simulink model "PCM"  (R2019b)
settings: Solver=FixedStepAuto  StartTime=0.0  StopTime=10.0  FixedStep=0.1  RelTol=1e-3
settings Model: Creator=JDALUZ1  LastModifiedBy=EMORAI12
settings DebuggingCC: ArithmeticOperatorsInVariantConditions=warning
settings SFSimCC: CustomCodeUndefinedFunction=UseInterfaceOnly
settings CodeAppCC: StateflowObjectComments=on

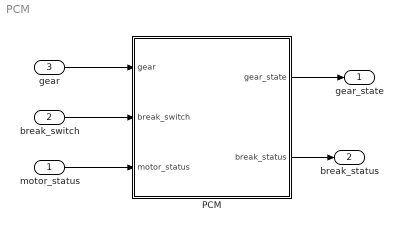
== system PCM ==
  motor_status : Inport
  break_switch : Inport  Port=2
  gear : Inport  Port=3
  PCM : Stateflow chart  TreatAsAtomicUnit=on
  gear_state : Outport
  break_status : Outport  Port=2
  wires:
  PCM/1(gear_state) -> gear_state/1
  PCM/2(break_status) -> break_status/1
  motor_status/1 -> PCM/3(motor_status)
  break_switch/1 -> PCM/2(break_switch)
  gear/1 -> PCM/1(gear)

== stateflow chart PCM/PCM ==
  state checking_GSM_state
    entry:
    gear_state=0;
    during:
    if(gear==0)
    gear_state=0;
    elseif(gear==1)
    gear_state=1;
    elseif(gear==2)
    gear_state=2;
    elseif(gear==3)
    gear_state=3;
    elseif(gear==4)
    gear_state=4;
    end
    aux_1=0;
  state motor_off_no_gear_change
    entry:
    break_status=0;
    break_status=break_switch;%atribui o estado do freio
    gear_state = 1; %não atribui o estado da marcha
    aux_1=1;
  state motor_on_gear_change_enable
    entry:
    break_status=break_switch;
    gear_state=gear;
    during:
    break_status=break_switch;%atribui o estado do freio
    gear_state=gear;%atribui o estado da marcha
    aux_1=1;
  (default) -> checking_GSM_state
  motor_off_no_gear_change -> motor_off_no_gear_change [order 1] : [motor_status==0]
  motor_on_gear_change_enable -> motor_on_gear_change_enable [order 1] : [motor_status==1]
  checking_GSM_state -> motor_off_no_gear_change [order 1] : [motor_status==0 && aux_1==0]
  checking_GSM_state -> motor_on_gear_change_enable [order 2] : [motor_status==1&& aux_1==0]
  motor_off_no_gear_change -> checking_GSM_state [order 2] : [motor_status==1 && aux_1==1 && gear_state ==1]
  motor_on_gear_change_enable -> checking_GSM_state [order 2] : [motor_status==0 && aux_1==1]
  data: gear input; gear_state output; break_switch input; break_status output; motor_status input; aux_1 local
